simulink model "accumulator"  (R2020b)
settings: Solver=FixedStepDiscrete  StartTime=0.0  StopTime=stopTime  FixedStep=2.0833333333333333e-05  RelTol=1e-3
libraries: hdlsllib x5
settings Model: Creator=Ross  LastModifiedBy=tyler
settings DataIOCC: SaveOutput=off  SaveTime=off  ReturnWorkspaceOutputs=off
settings OptimizationCC: BlockReduction=off  ConditionallyExecuteInputs=off  DefaultParameterBehavior=Inlined
settings DebuggingCC: ReadBeforeWriteMsg=DisableAll  WriteAfterWriteMsg=DisableAll  WriteAfterReadMsg=DisableAll  AlgebraicLoopMsg=error  MultiTaskDSMMsg=none  SingleTaskRateTransMsg=error  PregeneratedLibrarySubsystemCodeDiagnostic=none  ArithmeticOperatorsInVariantConditions=warning
settings HardwareCC: ProdBitPerPointer=32  ProdBitPerSizeT=32  ProdBitPerPtrDiffT=32  ProdLargestAtomicFloat=None  ProdIntDivRoundTo=Undefined  ProdEndianess=Unspecified  ProdWordSize=32  ProdHWDeviceType=ASIC/FPGA->ASIC/FPGA  TargetBitPerPointer=64  TargetBitPerSizeT=64  TargetBitPerPtrDiffT=64  TargetLongLongMode=on  TargetIntDivRoundTo=Zero  TargetEndianess=LittleEndian  TargetWordSize=64  TargetHWDeviceType=Custom Processor->MATLAB Host Computer  ProdEqTarget=off
settings ModelReferenceCC: UpdateModelReferenceTargets=IfOutOfDate
settings SFSimCC: SFSimEcho=off  SimUseLocalCustomCode=off  CustomCodeUndefinedFunction=UseInterfaceOnly
settings RTWCC: RTWUseLocalCustomCode=off

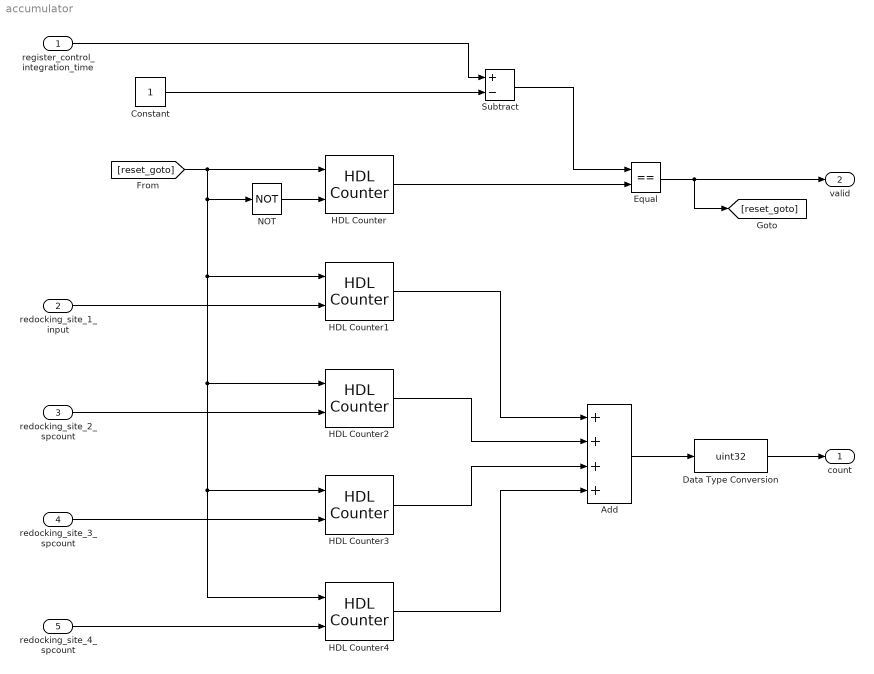
== system accumulator ==
  register_control_integration_time : Inport  OutDataTypeStr=uint32  PortDimensions=1  SampleTime=[2.0833333333333333e-05,0]
  redocking_site_1_input : Inport  Port=2  OutDataTypeStr=boolean  PortDimensions=[1 1]  SampleTime=[2.0833333333333333e-05,0]
  redocking_site_2_spcount : Inport  Port=3  OutDataTypeStr=boolean  PortDimensions=[1 1]  SampleTime=[2.0833333333333333e-05,0]
  redocking_site_3_spcount : Inport  Port=4  OutDataTypeStr=boolean  PortDimensions=[1 1]  SampleTime=[2.0833333333333333e-05,0]
  redocking_site_4_spcount : Inport  Port=5  OutDataTypeStr=boolean  PortDimensions=[1 1]  SampleTime=[2.0833333333333333e-05,0]
  Add : Sum  Inputs=++++
  Constant : Constant  OutDataTypeStr=uint32  SampleTime=-1
  Data Type Conversion : DataTypeConversion  OutDataTypeStr=uint32
  Equal : RelationalOperator  Operator===  OutDataTypeStr=boolean  RndMeth=Simplest
  HDL Counter{,1..4} (5 alike) : hdlsllib/Sources/HDL Counter  CountType=Count limited  CountInit=0  CountStep=1  CountMax=1073741823  CountFromType=Initial value  CountFrom=0  CountResetPort=on  CountLoadPort=off  CountEnbPort=on  CountDirPort=off  CountDataType=Unsigned  CountWordLen=30  CountFracLen=0  CountSampTime=1
  NOT : Logic  Operator=NOT  IconShape=distinctive  AllPortsSameDT=off  OutDataTypeStr=boolean
  Subtract : Sum  Inputs=+-
  count : Outport  OutDataTypeStr=fixdt(0,18,0)  PortDimensions=1  SampleTime=[2.0833333333333333e-05,0]
  valid : Outport  Port=2  OutDataTypeStr=boolean  PortDimensions=1  SampleTime=[2.0833333333333333e-05,0]
  wires:
  Equal/1 -> [reset_goto], valid/1
  HDL Counter/1 -> Equal/2
  [reset_goto] -> HDL Counter1/1, HDL Counter2/1, HDL Counter4/1, HDL Counter3/1, NOT/1, HDL Counter/1
  NOT/1 -> HDL Counter/2
  redocking_site_1_input/1 -> HDL Counter1/2
  redocking_site_2_spcount/1 -> HDL Counter2/2
  redocking_site_3_spcount/1 -> HDL Counter3/2
  HDL Counter2/1 -> Add/2
  HDL Counter3/1 -> Add/3
  HDL Counter4/1 -> Add/4
  HDL Counter1/1 -> Add/1
  redocking_site_4_spcount/1 -> HDL Counter4/2
  Subtract/1 -> Equal/1
  Constant/1 -> Subtract/2
  register_control_integration_time/1 -> Subtract/1
  Add/1 -> Data Type Conversion/1
  Data Type Conversion/1 -> count/1
